simulink model "motor_model_updated"  (R2020a)
settings: Solver=ode1  StartTime=0.0  StopTime=inf  FixedStep=0.0001  RelTol=1e-3  EnableMultiTasking=on
libraries: arduinolib x7
settings Model: SimulationMode=external  SILPILModeSetting=veronly  ExtModeTrigDuration=2  Creator=Ninad  LastModifiedBy=gdube
settings DataIOCC: LimitDataPoints=on  SaveFormat=Array  ReturnWorkspaceOutputs=off
settings OptimizationCC: BlockReduction=off  EnhancedBackFolding=on  PassReuseOutputArgsAs=Individual arguments  ExpressionDepthLimit=2147483647  ZeroExternalMemoryAtStartup=off  ZeroInternalMemoryAtStartup=off  MaxStackSize=64  OptimizeBlockOrder=speed  DifferentSizesBufferReuse=on  OptimizationCustomize=off  EfficientTunableParamExpr=on
settings DebuggingCC: UnderspecifiedInitializationDetection=Classic  MergeDetectMultiDrivingBlocksExec=none  SolverPrmCheckMsg=warning  ParameterTunabilityLossMsg=error  FcnCallInpInsideContextMsg=warning  StateNameClashWarn=warning  SFUnexpectedBacktrackingDiag=warning  SFNoUnconditionalDefaultTransitionDiag=warning  SFExecutionAtInitializationDiag=none  ArithmeticOperatorsInVariantConditions=warning
settings HardwareCC: ProdBitPerInt=16  ProdBitPerPointer=16  ProdBitPerSizeT=16  ProdBitPerPtrDiffT=16  ProdLargestAtomicFloat=None  ProdWordSize=8  ProdHWDeviceType=Atmel->AVR  UseEmbeddedCoderFeatures=off
settings ModelReferenceCC: PropagateSignalLabelsOutOfModel=off
settings SFSimCC: SimUseLocalCustomCode=off  MATLABDynamicMemAlloc=off  CustomCodeUndefinedFunction=UseInterfaceOnly
settings RTWCC: SystemTargetFile=ert.tlc  HardwareBoard=Arduino Mega 2560  TLCOptions=-aInlineSetEventsForThisBaseRateFcn=TLC_FALSE -aSuppressMultiTaskScheduler=TLC_FALSE -aRateBasedStepFcn=1  TemplateMakefile=ert_default_tmf  RTWUseLocalCustomCode=off  Toolchain=Arduino AVR  BuildConfiguration=Faster Runs  CodeExecutionProfiling=on
settings CodeAppCC: ForceParamTrailComments=on  IgnoreCustomStorageClasses=off  OperatorAnnotations=on  SimulinkDataObjDesc=on  SFDataObjDesc=on  InsertBlockDesc=on
settings ERTTargetCC: SupportContinuousTime=on  SupportNonInlinedSFcns=on  SupportVariableSizeSignals=on  ExtModeStaticAllocSize=2048
settings ConfigComp: CovMetricSettings=dw  CovHtmlReporting=on  CovSaveCumulativeToWorkspaceVar=on  CovSaveSingleToWorkspaceVar=on  CovExternalEMLEnable=off  CovSFcnEnable=off

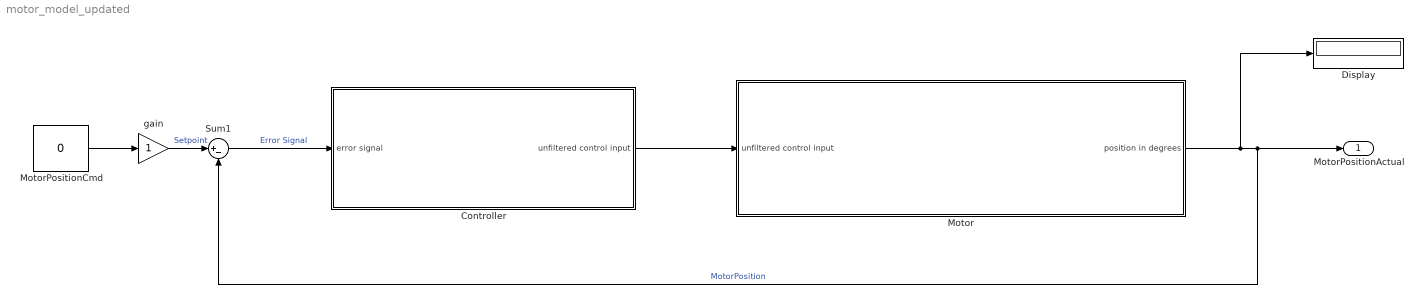
== system motor_model_updated ==
  Controller : Subsystem
  Display : Display
  Motor : Subsystem
  MotorPositionCmd : Constant  Value=0
  Sum1 : Sum  Inputs=|+-
  gain : Gain
  MotorPositionActual : Outport  VectorParamsAs1DForOutWhenUnconnected=off
  wires:
  gain/1 -> Sum1/1  "Setpoint"
  MotorPositionCmd/1 -> gain/1
  Motor/1(position in degrees) -> Display/1, MotorPositionActual/1, Sum1/2  "MotorPosition"
  Controller/1(unfiltered control input) -> Motor/1(unfiltered control input)
  Sum1/1 -> Controller/1(error signal)  "Error Signal"

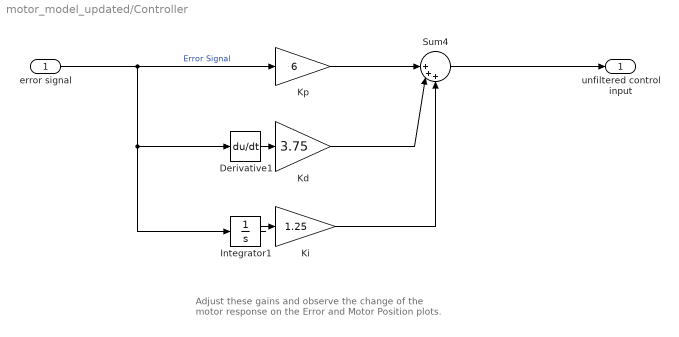
== system motor_model_updated/Controller ==
  note: Adjust these gains and observe the change of the
      | motor response on the Error and Motor Position
      | plots.
  error signal : Inport
  Derivative1 : Derivative
  Integrator1 : Integrator
  Kd : Gain  Gain=3.75
  Ki : Gain  Gain=1.25
  Kp : Gain  Gain=6
  Sum4 : Sum  Inputs=||+++
  unfiltered control input : Outport
  wires:
  Kd/1 -> Sum4/2
  Integrator1/1 -> Ki/1
  Ki/1 -> Sum4/3
  Derivative1/1 -> Kd/1
  error signal/1 -> Derivative1/1, Integrator1/1, Kp/1  "Error Signal"
  Kp/1 -> Sum4/1
  Sum4/1 -> unfiltered control input/1

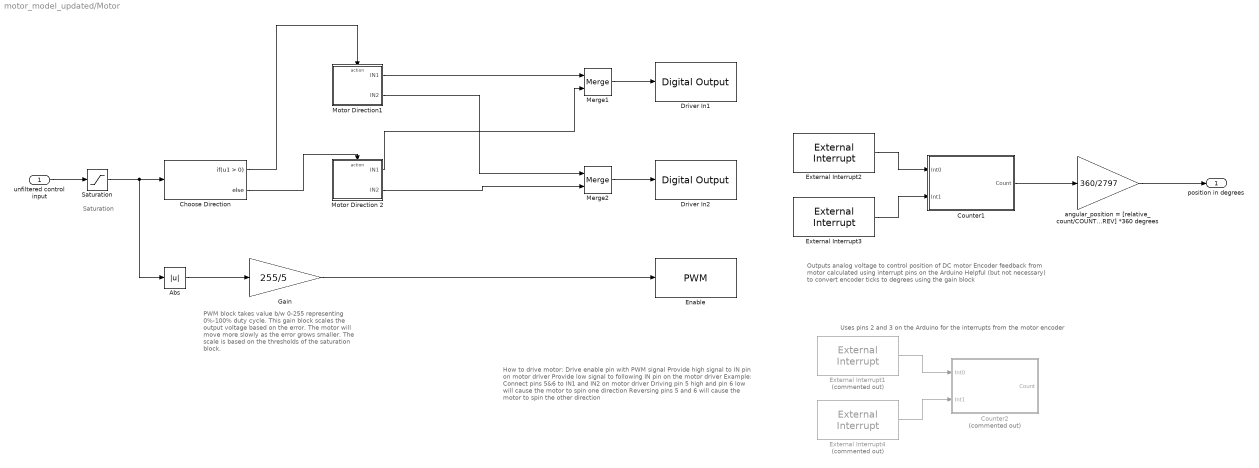
== system motor_model_updated/Motor ==
  note: PWM block takes value b/w 0-255 representing
      | 0%-100% duty cycle. This gain block scales the
      | output voltage based on the error. The motor will
      | move more slowly as the error grows
      | smaller. The scale is based on the thresholds
      | of the saturation block.
  note: Outputs analog voltage to control position of DC motor
      |
      | Encoder feedback from motor calculated using interrupt pins on the Arduino
      |
      | Helpful (but not necessary) to convert encoder ticks to degrees using the
      | gain block
  note: Saturation
  note: How to drive motor:
      | Drive enable pin with PWM signal
      | Provide high signal to IN pin on motor driver
      | Provide low signal to following IN pin on the motor driver
      |
      | Example:
      | Connect pins 5&6 to IN1 and IN2 on motor driver
      | Driving pin 5 high and pin 6 low will cause the motor to spin one direction
      | Reversing pins 5 and 6 will cause the motor to spin the other direction
  note: Uses pins 2 and 3 on the Arduino for the interrupts from the motor encoder
  unfiltered control input : Inport
  Abs : Abs
  Choose Direction : If
  Counter1 : Subsystem
  Counter2 : Subsystem  Commented=on
  Driver In1 : arduinolib/Digital Output  pinNumber=30  Direction=output  blockPlatform=arduino
  Driver In2 : arduinolib/Digital Output  pinNumber=31  Direction=output  blockPlatform=arduino
  Enable : arduinolib/PWM  pinNumber=5  frequencyType=Default  desiredFrequency=490.2  achievableFrequency=490.2
  External Interrupt1 : arduinolib/External Interrupt  Commented=on  Pin=2  PullUp=on  Mode=CHANGE  InterruptSimulationInput=off
      settings: SourceProductBaseCode=ARDUINO
  External Interrupt2 : arduinolib/External Interrupt  Pin=2  PullUp=on  Mode=CHANGE  InterruptSimulationInput=off
      settings: SourceProductBaseCode=ARDUINO
  External Interrupt3 : arduinolib/External Interrupt  Pin=3  PullUp=on  Mode=CHANGE  InterruptSimulationInput=off
      settings: SourceProductBaseCode=ARDUINO
  External Interrupt4 : arduinolib/External Interrupt  Commented=on  Pin=3  PullUp=on  Mode=CHANGE  InterruptSimulationInput=off
      settings: SourceProductBaseCode=ARDUINO
  Gain : Gain  Gain=255/5
  Merge1 : Merge
  Merge2 : Merge
  Motor Direction 2 : Subsystem  TreatAsAtomicUnit=on
  Motor Direction1 : Subsystem  TreatAsAtomicUnit=on
  Saturation : Saturate  UpperLimit=5  LowerLimit=-5
  angular_position = [relative_count/COUNTS_PER_REV] *360 degrees : Gain  Gain=360/2797
  position in degrees : Outport  VectorParamsAs1DForOutWhenUnconnected=off
  wires:
  angular_position = [relative_count/COUNTS_PER_REV] *360 degrees/1 -> position in degrees/1
  unfiltered control input/1 -> Saturation/1
  Counter1/1(Count) -> angular_position = [relative_count/COUNTS_PER_REV] *360 degrees/1
  Saturation/1 -> Abs/1, Choose Direction/1
  Choose Direction/1 -> Motor Direction1/Action
  Choose Direction/2 -> Motor Direction 2/Action
  Motor Direction1/1(IN1) -> Merge1/1
  Motor Direction 2/1(IN1) -> Merge1/2
  Motor Direction1/2(IN2) -> Merge2/1
  Motor Direction 2/2(IN2) -> Merge2/2
  Abs/1 -> Gain/1
  Gain/1 -> Enable/1
  Merge1/1 -> Driver In1/1
  Merge2/1 -> Driver In2/1
  External Interrupt1/1 -> Counter2/1(Int0)
  External Interrupt4/1 -> Counter2/2(Int1)
  External Interrupt2/1 -> Counter1/1(Int0)
  External Interrupt3/1 -> Counter1/2(Int1)

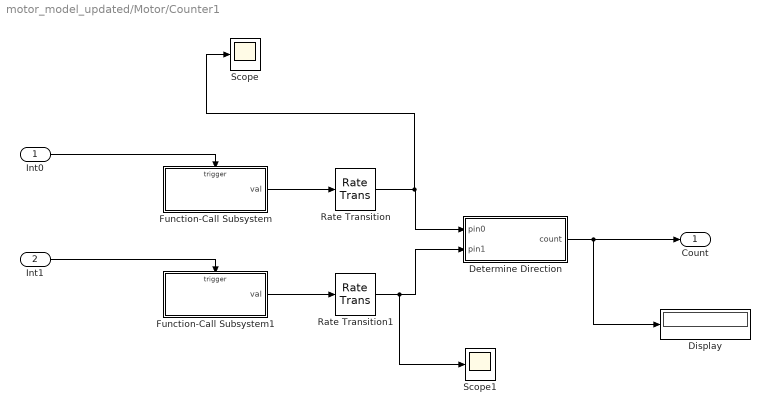
== system motor_model_updated/Motor/Counter1 ==
  Int0 : Inport
  Int1 : Inport  Port=2
  Determine Direction : Subsystem
  Display : Display
  Function-Call Subsystem : Subsystem  TreatAsAtomicUnit=on
  Function-Call Subsystem1 : Subsystem  TreatAsAtomicUnit=on
  Rate Transition : RateTransition  Deterministic=off
  Rate Transition1 : RateTransition  Deterministic=off
  Scope : Scope
  Scope1 : Scope
  Count : Outport
  wires:
  Function-Call Subsystem/1(val) -> Rate Transition/1
  Function-Call Subsystem1/1(val) -> Rate Transition1/1
  Int0/1 -> Function-Call Subsystem/Trigger
  Int1/1 -> Function-Call Subsystem1/Trigger
  Rate Transition/1 -> Scope/1, Determine Direction/1(pin0)
  Rate Transition1/1 -> Scope1/1, Determine Direction/2(pin1)
  Determine Direction/1(count) -> Display/1, Count/1

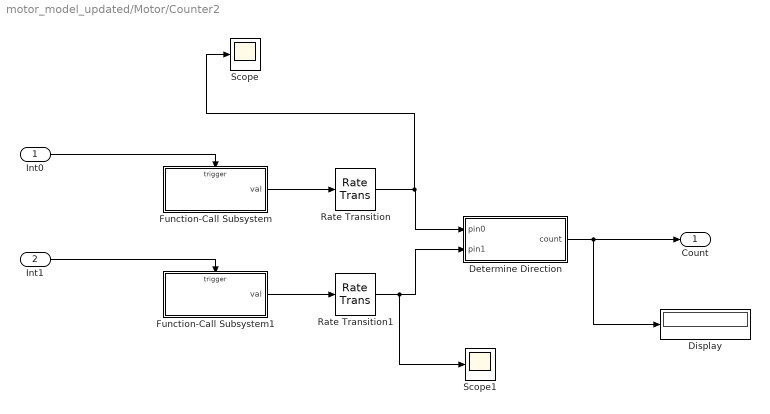
== system motor_model_updated/Motor/Counter2 ==
  Int0 : Inport
  Int1 : Inport  Port=2
  Determine Direction : Subsystem
  Display : Display
  Function-Call Subsystem : Subsystem  TreatAsAtomicUnit=on
  Function-Call Subsystem1 : Subsystem  TreatAsAtomicUnit=on
  Rate Transition : RateTransition  Deterministic=off
  Rate Transition1 : RateTransition  Deterministic=off
  Scope : Scope
  Scope1 : Scope
  Count : Outport
  wires:
  Function-Call Subsystem/1(val) -> Rate Transition/1
  Function-Call Subsystem1/1(val) -> Rate Transition1/1
  Int0/1 -> Function-Call Subsystem/Trigger
  Int1/1 -> Function-Call Subsystem1/Trigger
  Rate Transition/1 -> Scope/1, Determine Direction/1(pin0)
  Rate Transition1/1 -> Scope1/1, Determine Direction/2(pin1)
  Determine Direction/1(count) -> Display/1, Count/1

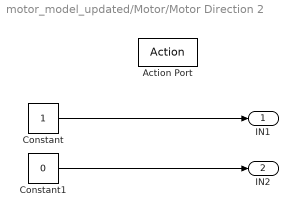
== system motor_model_updated/Motor/Motor Direction 2 ==
  Action Port : ActionPort  ActionPortLabel=else
  Constant : Constant
  Constant1 : Constant  Value=0
  IN1 : Outport
  IN2 : Outport  Port=2
  wires:
  Constant/1 -> IN1/1
  Constant1/1 -> IN2/1

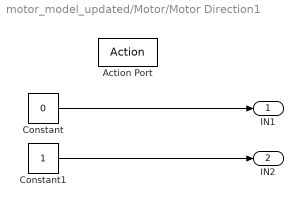
== system motor_model_updated/Motor/Motor Direction1 ==
  Action Port : ActionPort  ActionPortLabel=if(u1 > 0)
  Constant : Constant  Value=0
  Constant1 : Constant
  IN1 : Outport
  IN2 : Outport  Port=2
  wires:
  Constant/1 -> IN1/1
  Constant1/1 -> IN2/1

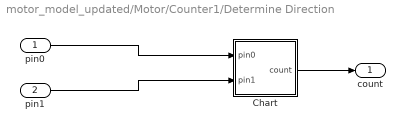
== system motor_model_updated/Motor/Counter1/Determine Direction ==
  pin0 : Inport
  pin1 : Inport  Port=2
  Chart : Stateflow chart  TreatAsAtomicUnit=on
  count : Outport
  wires:
  pin0/1 -> Chart/1(pin0)
  pin1/1 -> Chart/2(pin1)
  Chart/1(count) -> count/1

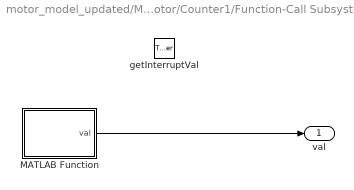
== system motor_model_updated/Motor/Counter1/Function-Call Subsystem ==
  getInterruptVal : TriggerPort  TriggerType=function-call  VariantControl=Variant
  MATLAB Function : MATLAB Function  TreatAsAtomicUnit=on
  val : Outport
  wires:
  MATLAB Function/1(val) -> val/1

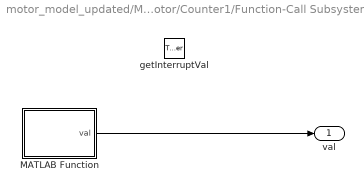
== system motor_model_updated/Motor/Counter1/Function-Call Subsystem1 ==
  getInterruptVal : TriggerPort  TriggerType=function-call  VariantControl=Variant
  MATLAB Function : MATLAB Function  TreatAsAtomicUnit=on
  val : Outport
  wires:
  MATLAB Function/1(val) -> val/1

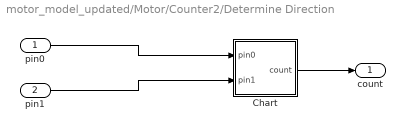
== system motor_model_updated/Motor/Counter2/Determine Direction ==
  pin0 : Inport
  pin1 : Inport  Port=2
  Chart : Stateflow chart  TreatAsAtomicUnit=on
  count : Outport
  wires:
  pin0/1 -> Chart/1(pin0)
  pin1/1 -> Chart/2(pin1)
  Chart/1(count) -> count/1

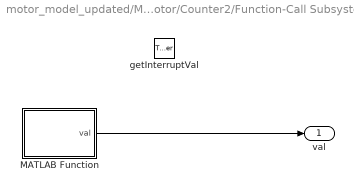
== system motor_model_updated/Motor/Counter2/Function-Call Subsystem ==
  getInterruptVal : TriggerPort  TriggerType=function-call  VariantControl=Variant
  MATLAB Function : MATLAB Function  TreatAsAtomicUnit=on
  val : Outport
  wires:
  MATLAB Function/1(val) -> val/1

== system motor_model_updated/Motor/Counter2/Function-Call Subsystem1 ==
  getInterruptVal : TriggerPort  TriggerType=function-call  VariantControl=Variant
  MATLAB Function : MATLAB Function  TreatAsAtomicUnit=on
  val : Outport
  wires:
  MATLAB Function/1(val) -> val/1

== stateflow chart motor_model_updated/Motor/Counter2/Determine Direction/Chart ==
  state State01
  state State00
  state State11
  state State10
  State01 -> State00 [order 1] : [pin0==0]{count = count - 1;}
  State01 -> State11 [order 2] : [pin1==1]{count = count + 1;}
  (default) -> State00
  State00 -> State01 [order 2] : [pin0==1]{count = count + 1;}
  State11 -> State01 [order 1] : [pin1==0]{count = count - 1;}
  State11 -> State10 [order 2] : [pin0==0]{count = count + 1;}
  State00 -> State10 [order 1] : [pin1==1]{count = count - 1;}
  State10 -> State00 [order 1] : [pin1==0]{count = count + 1;}
  State10 -> State11 [order 2] : [pin0==1]{count = count - 1;}
  data: pin0 input; pin1 input; count output =0

== matlab function motor_model_updated/Motor/Counter2/Function-Call Subsystem/MATLAB Function ==
  data: val output
function val = readPinValue()

a = arduino;
u = readDigitalPin(a, 'D2');

val = u;

== matlab function motor_model_updated/Motor/Counter2/Function-Call Subsystem1/MATLAB Function ==
  data: val output
function val = readPinValue()

a = arduino;
u = readDigitalPin(a, 'D3');

val = u;

== stateflow chart motor_model_updated/Motor/Counter1/Determine Direction/Chart ==
  state State01
  state State00
  state State11
  state State10
  State01 -> State00 [order 1] : [pin0==0]{count = count - 1;}
  State01 -> State11 [order 2] : [pin1==1]{count = count + 1;}
  (default) -> State00
  State00 -> State01 [order 2] : [pin0==1]{count = count + 1;}
  State11 -> State01 [order 1] : [pin1==0]{count = count - 1;}
  State11 -> State10 [order 2] : [pin0==0]{count = count + 1;}
  State00 -> State10 [order 1] : [pin1==1]{count = count - 1;}
  State10 -> State00 [order 1] : [pin1==0]{count = count + 1;}
  State10 -> State11 [order 2] : [pin0==1]{count = count - 1;}
  data: pin0 input; pin1 input; count output =0

== matlab function motor_model_updated/Motor/Counter1/Function-Call Subsystem/MATLAB Function ==
  data: val output
function val = readPinValue()

a = arduino;
u = readDigitalPin(a, 'D2');

val = u;

== matlab function motor_model_updated/Motor/Counter1/Function-Call Subsystem1/MATLAB Function ==
  data: val output
function val = readPinValue()

a = arduino;
u = readDigitalPin(a, 'D3');

val = u;
